simulink model "sound_effects"  (R2020b)
settings: Solver=FixedStepDiscrete  StartTime=0.0  StopTime=stopTime  RelTol=1e-3
PreLoadFcn:
  | addpath('../simple_gain_vector')
  | addpath('../flanger')
  | addpath('../bitcrusher')
  | addpath('../echo')
InitFcn:
  | initCallback
StopFcn:
  | stopCallback
undefined symbols (not defined in the file or in its folder): mp
settings Model: DataTypeOverride=Off  Creator=Ross  LastModifiedBy=wickh
settings SolverCC: AutoInsertRateTranBlk=on
settings DataIOCC: ReturnWorkspaceOutputs=off
settings OptimizationCC: BlockReduction=off  ConditionallyExecuteInputs=off  DefaultParameterBehavior=Inlined
settings DebuggingCC: SignalInfNanChecking=error  SignalRangeChecking=warning  ReadBeforeWriteMsg=DisableAll  WriteAfterWriteMsg=DisableAll  WriteAfterReadMsg=DisableAll  AlgebraicLoopMsg=error  MultiTaskDSMMsg=none  SingleTaskRateTransMsg=error  ParameterUnderflowMsg=warning  UnderSpecifiedDataTypeMsg=error  PregeneratedLibrarySubsystemCodeDiagnostic=none  ArithmeticOperatorsInVariantConditions=warning
settings HardwareCC: ProdBitPerPointer=32  ProdBitPerSizeT=32  ProdBitPerPtrDiffT=32  ProdLargestAtomicFloat=None  ProdIntDivRoundTo=Undefined  ProdEndianess=Unspecified  ProdWordSize=32  ProdHWDeviceType=ASIC/FPGA->ASIC/FPGA  TargetBitPerPointer=64  TargetBitPerSizeT=64  TargetBitPerPtrDiffT=64  TargetLongLongMode=on  TargetIntDivRoundTo=Zero  TargetEndianess=LittleEndian  TargetWordSize=64  TargetHWDeviceType=Custom Processor->MATLAB Host Computer  ProdEqTarget=off
settings ModelReferenceCC: UpdateModelReferenceTargets=IfOutOfDate
settings SFSimCC: SFSimEcho=off  SimUseLocalCustomCode=off  CustomCodeUndefinedFunction=UseInterfaceOnly
settings RTWCC: RTWUseLocalCustomCode=off

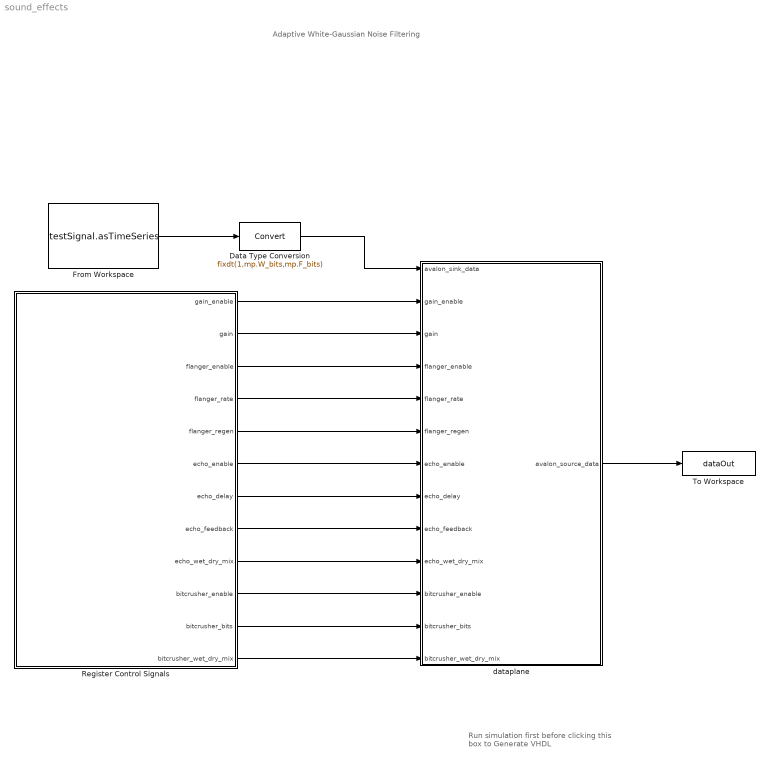
== system sound_effects ==
  note: Adaptive White-Gaussian Noise Filtering
  note: Run simulation first
      | before clicking this box to
      | Generate VHDL
  Data Type Conversion : DataTypeConversion  OutDataTypeStr=fixdt(1,mp.W_bits,mp.F_bits)
  From Workspace : FromWorkspace  VariableName=testSignal.asTimeSeries  OutDataTypeStr=double  SampleTime=mp.Ts_sim  Interpolate=off  OutputAfterFinalValue=Setting to zero
  Register Control Signals : Subsystem
  To Workspace : ToWorkspace  VariableName=dataOut  SaveFormat=Timeseries  SampleTime=-1
      settings: Save2DSignal=2-D array (concatenate along first dimension)
  dataplane : Subsystem  TreatAsAtomicUnit=on
  wires:
  dataplane/1(avalon_source_data) -> To Workspace/1
  From Workspace/1 -> Data Type Conversion/1
  Data Type Conversion/1 -> dataplane/1(avalon_sink_data)
  Register Control Signals/1(gain_enable) -> dataplane/2(gain_enable)
  Register Control Signals/2(gain) -> dataplane/3(gain)
  Register Control Signals/3(flanger_enable) -> dataplane/4(flanger_enable)
  Register Control Signals/4(flanger_rate) -> dataplane/5(flanger_rate)
  Register Control Signals/5(flanger_regen) -> dataplane/6(flanger_regen)
  Register Control Signals/6(echo_enable) -> dataplane/7(echo_enable)
  Register Control Signals/7(echo_delay) -> dataplane/8(echo_delay)
  Register Control Signals/8(echo_feedback) -> dataplane/9(echo_feedback)
  Register Control Signals/9(echo_wet_dry_mix) -> dataplane/10(echo_wet_dry_mix)
  Register Control Signals/10(bitcrusher_enable) -> dataplane/11(bitcrusher_enable)
  Register Control Signals/11(bitcrusher_bits) -> dataplane/12(bitcrusher_bits)
  Register Control Signals/12(bitcrusher_wet_dry_mix) -> dataplane/13(bitcrusher_wet_dry_mix)

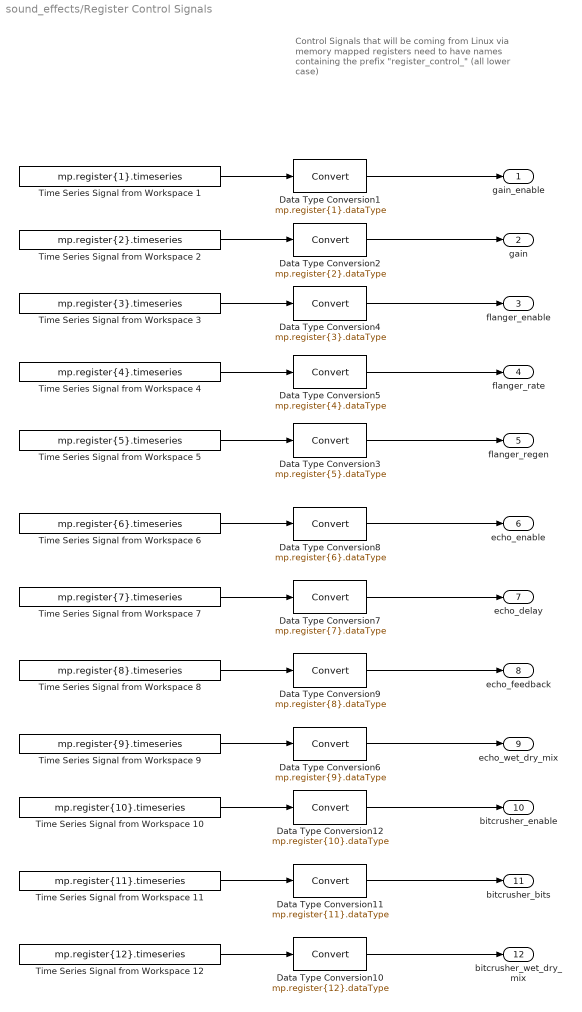
== system sound_effects/Register Control Signals ==
  note: Control Signals that will be coming from Linux via
      | memory mapped registers need to have names
      | containing the prefix "register_control_"
      | (all lower case)
  Data Type Conversion1 : DataTypeConversion  OutDataTypeStr=mp.register{1}.dataType
  Data Type Conversion10 : DataTypeConversion  OutDataTypeStr=mp.register{12}.dataType
  Data Type Conversion11 : DataTypeConversion  OutDataTypeStr=mp.register{11}.dataType
  Data Type Conversion12 : DataTypeConversion  OutDataTypeStr=mp.register{10}.dataType
  Data Type Conversion2 : DataTypeConversion  OutDataTypeStr=mp.register{2}.dataType
  Data Type Conversion3 : DataTypeConversion  OutDataTypeStr=mp.register{5}.dataType
  Data Type Conversion4 : DataTypeConversion  OutDataTypeStr=mp.register{3}.dataType
  Data Type Conversion5 : DataTypeConversion  OutDataTypeStr=mp.register{4}.dataType
  Data Type Conversion6 : DataTypeConversion  OutDataTypeStr=mp.register{9}.dataType
  Data Type Conversion7 : DataTypeConversion  OutDataTypeStr=mp.register{7}.dataType
  Data Type Conversion8 : DataTypeConversion  OutDataTypeStr=mp.register{6}.dataType
  Data Type Conversion9 : DataTypeConversion  OutDataTypeStr=mp.register{8}.dataType
  Time Series Signal from Workspace 1 : FromWorkspace  VariableName=mp.register{1}.timeseries  OutDataTypeStr=double  SampleTime=mp.Ts_sim
  Time Series Signal from Workspace 10 : FromWorkspace  VariableName=mp.register{10}.timeseries  OutDataTypeStr=double  SampleTime=mp.Ts_sim
  Time Series Signal from Workspace 11 : FromWorkspace  VariableName=mp.register{11}.timeseries  OutDataTypeStr=double  SampleTime=mp.Ts_sim
  Time Series Signal from Workspace 12 : FromWorkspace  VariableName=mp.register{12}.timeseries  OutDataTypeStr=double  SampleTime=mp.Ts_sim
  Time Series Signal from Workspace 2 : FromWorkspace  VariableName=mp.register{2}.timeseries  OutDataTypeStr=double  SampleTime=mp.Ts_sim
  Time Series Signal from Workspace 3 : FromWorkspace  VariableName=mp.register{3}.timeseries  OutDataTypeStr=double  SampleTime=mp.Ts_sim
  Time Series Signal from Workspace 4 : FromWorkspace  VariableName=mp.register{4}.timeseries  OutDataTypeStr=double  SampleTime=mp.Ts_sim
  Time Series Signal from Workspace 5 : FromWorkspace  VariableName=mp.register{5}.timeseries  OutDataTypeStr=double  SampleTime=mp.Ts_sim
  Time Series Signal from Workspace 6 : FromWorkspace  VariableName=mp.register{6}.timeseries  OutDataTypeStr=double  SampleTime=mp.Ts_sim
  Time Series Signal from Workspace 7 : FromWorkspace  VariableName=mp.register{7}.timeseries  OutDataTypeStr=double  SampleTime=mp.Ts_sim
  Time Series Signal from Workspace 8 : FromWorkspace  VariableName=mp.register{8}.timeseries  OutDataTypeStr=double  SampleTime=mp.Ts_sim
  Time Series Signal from Workspace 9 : FromWorkspace  VariableName=mp.register{9}.timeseries  OutDataTypeStr=double  SampleTime=mp.Ts_sim
  gain_enable : Outport  VectorParamsAs1DForOutWhenUnconnected=off
  gain : Outport  Port=2  VectorParamsAs1DForOutWhenUnconnected=off
  flanger_enable : Outport  Port=3  VectorParamsAs1DForOutWhenUnconnected=off
  flanger_rate : Outport  Port=4  VectorParamsAs1DForOutWhenUnconnected=off
  flanger_regen : Outport  Port=5  VectorParamsAs1DForOutWhenUnconnected=off
  echo_enable : Outport  Port=6  VectorParamsAs1DForOutWhenUnconnected=off
  echo_delay : Outport  Port=7  VectorParamsAs1DForOutWhenUnconnected=off
  echo_feedback : Outport  Port=8  VectorParamsAs1DForOutWhenUnconnected=off
  echo_wet_dry_mix : Outport  Port=9  VectorParamsAs1DForOutWhenUnconnected=off
  bitcrusher_enable : Outport  Port=10  VectorParamsAs1DForOutWhenUnconnected=off
  bitcrusher_bits : Outport  Port=11  VectorParamsAs1DForOutWhenUnconnected=off
  bitcrusher_wet_dry_mix : Outport  Port=12  VectorParamsAs1DForOutWhenUnconnected=off
  wires:
  Time Series Signal from Workspace 1/1 -> Data Type Conversion1/1
  Data Type Conversion1/1 -> gain_enable/1
  Time Series Signal from Workspace 2/1 -> Data Type Conversion2/1
  Data Type Conversion2/1 -> gain/1
  Data Type Conversion4/1 -> flanger_enable/1
  Data Type Conversion3/1 -> flanger_regen/1
  Data Type Conversion5/1 -> flanger_rate/1
  Time Series Signal from Workspace 5/1 -> Data Type Conversion3/1
  Time Series Signal from Workspace 3/1 -> Data Type Conversion4/1
  Time Series Signal from Workspace 4/1 -> Data Type Conversion5/1
  Data Type Conversion9/1 -> echo_feedback/1
  Data Type Conversion6/1 -> echo_wet_dry_mix/1
  Time Series Signal from Workspace 8/1 -> Data Type Conversion9/1
  Data Type Conversion8/1 -> echo_enable/1
  Time Series Signal from Workspace 9/1 -> Data Type Conversion6/1
  Data Type Conversion7/1 -> echo_delay/1
  Time Series Signal from Workspace 6/1 -> Data Type Conversion8/1
  Time Series Signal from Workspace 7/1 -> Data Type Conversion7/1
  Data Type Conversion12/1 -> bitcrusher_enable/1
  Time Series Signal from Workspace 10/1 -> Data Type Conversion12/1
  Time Series Signal from Workspace 12/1 -> Data Type Conversion10/1
  Data Type Conversion11/1 -> bitcrusher_bits/1
  Data Type Conversion10/1 -> bitcrusher_wet_dry_mix/1
  Time Series Signal from Workspace 11/1 -> Data Type Conversion11/1

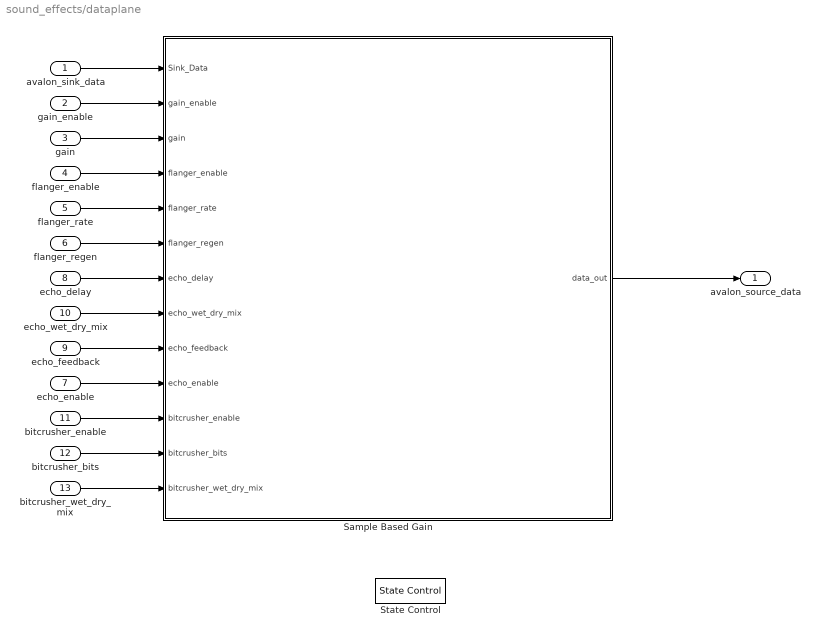
== system sound_effects/dataplane ==
  avalon_sink_data : Inport
  gain_enable : Inport  Port=2
  gain : Inport  Port=3
  flanger_enable : Inport  Port=4
  flanger_rate : Inport  Port=5
  flanger_regen : Inport  Port=6
  echo_enable : Inport  Port=7
  echo_delay : Inport  Port=8
  echo_feedback : Inport  Port=9
  echo_wet_dry_mix : Inport  Port=10
  bitcrusher_enable : Inport  Port=11
  bitcrusher_bits : Inport  Port=12
  bitcrusher_wet_dry_mix : Inport  Port=13
  Sample Based Gain : Subsystem
  State Control : StateControl  StateControl=Synchronous
  avalon_source_data : Outport  VectorParamsAs1DForOutWhenUnconnected=off
  wires:
  Sample Based Gain/1(data_out) -> avalon_source_data/1
  gain_enable/1 -> Sample Based Gain/2(gain_enable)
  avalon_sink_data/1 -> Sample Based Gain/1(Sink_Data)
  gain/1 -> Sample Based Gain/3(gain)
  flanger_enable/1 -> Sample Based Gain/4(flanger_enable)
  flanger_rate/1 -> Sample Based Gain/5(flanger_rate)
  flanger_regen/1 -> Sample Based Gain/6(flanger_regen)
  echo_feedback/1 -> Sample Based Gain/9(echo_feedback)
  echo_enable/1 -> Sample Based Gain/10(echo_enable)
  echo_wet_dry_mix/1 -> Sample Based Gain/8(echo_wet_dry_mix)
  echo_delay/1 -> Sample Based Gain/7(echo_delay)
  bitcrusher_enable/1 -> Sample Based Gain/11(bitcrusher_enable)
  bitcrusher_bits/1 -> Sample Based Gain/12(bitcrusher_bits)
  bitcrusher_wet_dry_mix/1 -> Sample Based Gain/13(bitcrusher_wet_dry_mix)

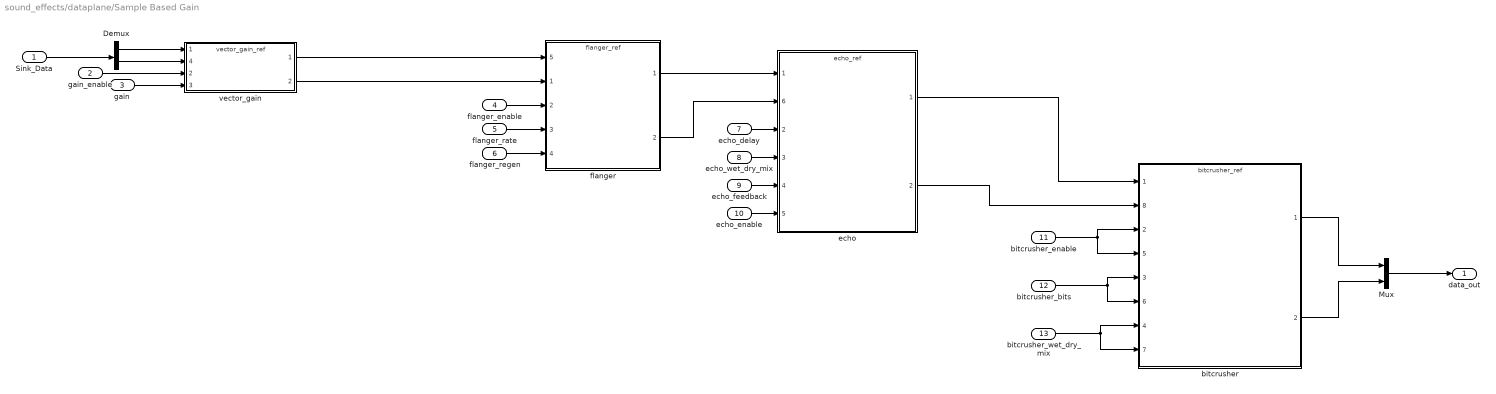
== system sound_effects/dataplane/Sample Based Gain ==
  Sink_Data : Inport
  gain_enable : Inport  Port=2
  gain : Inport  Port=3
  flanger_enable : Inport  Port=4
  flanger_rate : Inport  Port=5
  flanger_regen : Inport  Port=6
  echo_delay : Inport  Port=7
  echo_wet_dry_mix : Inport  Port=8
  echo_feedback : Inport  Port=9
  echo_enable : Inport  Port=10
  bitcrusher_enable : Inport  Port=11
  bitcrusher_bits : Inport  Port=12
  bitcrusher_wet_dry_mix : Inport  Port=13
  Demux : Demux  Outputs=2
  Mux : Mux  Inputs=2
  bitcrusher : ModelReference  ModelNameDialog=bitcrusher_ref  SimulationMode=Normal  ModelReferenceVersion=3.10
      settings: PortSchema="{\"entries\":[{\"content\":{\"sides\":[{\"content\":{\"connectorIds\":[\"In1\",\"In8\",\"In2\",\"In5\",\"In3\",\"In6\",\"In4\",\"In7\"]},\"type\":\"ConnectorPlacement.EquallySpacedRectSide\",\"uuid\":\"90c15296-b05c-4084-9131-8d1d83a85f81\"},{\"content\":{\"connectorIds\":[\"Out1\",\"Out2\"],\"side\":\"RIGHT\"},\"type\":\"ConnectorPlacement.EquallySpacedRectSide\",\"uuid\":\"9a8bffd3-a422-4815-8844-880c14b7d0b0\"},{\"content\":{\"connectorIds\":[],\"side\":\"TOP\"},\"type\":\"ConnectorPlacement.EquallySpacedRectSide\",\"uuid\":\"96339341-ea10-4881-8e29-794be7478c65\"},{\"content\":{\"connectorIds\":[],\"side\":\"HIDDEN\"},\"type\":\"ConnectorPlacement.EquallySpacedRectSide\",\"uuid\":\"4bb35bf2-de86-4de6-867a-84aa2bcf46f8\"}]},\"type\":\"ConnectorPlacement.EquallySpacedConnector\",\"uuid\":\"42256606-ddb3-4766-9977-bd7ae7f9f64f\"}],\"packageUris\":[\"http://schema.mathworks.com/mf0/Connector/R2020b\"],\"version\":\"1.0\"}"
  echo : ModelReference  ModelNameDialog=echo_ref  SimulationMode=Normal  ModelReferenceVersion=1.158
      settings: PortSchema="{\"entries\":[{\"content\":{\"sides\":[{\"content\":{\"connectorIds\":[\"In1\",\"In6\",\"In2\",\"In3\",\"In4\",\"In5\"]},\"type\":\"ConnectorPlacement.EquallySpacedRectSide\",\"uuid\":\"e306e1ad-d1b8-4582-952d-4c4191a99a81\"},{\"content\":{\"connectorIds\":[\"Out1\",\"Out2\"],\"side\":\"RIGHT\"},\"type\":\"ConnectorPlacement.EquallySpacedRectSide\",\"uuid\":\"8133f08a-39d0-44da-b52e-b96b1c72783c\"},{\"content\":{\"connectorIds\":[],\"side\":\"TOP\"},\"type\":\"ConnectorPlacement.EquallySpacedRectSide\",\"uuid\":\"327e31c7-8f91-4124-82a4-b2c62ce56765\"},{\"content\":{\"connectorIds\":[],\"side\":\"HIDDEN\"},\"type\":\"ConnectorPlacement.EquallySpacedRectSide\",\"uuid\":\"f85fe833-603d-4d04-9a61-60dde0930239\"}]},\"type\":\"ConnectorPlacement.EquallySpacedConnector\",\"uuid\":\"c6b2a458-4634-4ce8-98bc-50a2a0ff1bc4\"}],\"packageUris\":[\"http://schema.mathworks.com/mf0/Connector/R2020b\"],\"version\":\"1.0\"}"
  flanger : ModelReference  ModelNameDialog=flanger_ref  SimulationMode=Normal  ModelReferenceVersion=3.19
      settings: PortSchema="{\"entries\":[{\"content\":{\"sides\":[{\"content\":{\"connectorIds\":[\"In5\",\"In1\",\"In2\",\"In3\",\"In4\"]},\"type\":\"ConnectorPlacement.EquallySpacedRectSide\",\"uuid\":\"1d82ca4f-6eb6-4f28-946c-3ec85ec43cb1\"},{\"content\":{\"connectorIds\":[\"Out1\",\"Out2\"],\"side\":\"RIGHT\"},\"type\":\"ConnectorPlacement.EquallySpacedRectSide\",\"uuid\":\"239d2b31-0591-4f6b-b81b-3753802d9df9\"},{\"content\":{\"connectorIds\":[],\"side\":\"TOP\"},\"type\":\"ConnectorPlacement.EquallySpacedRectSide\",\"uuid\":\"6a0da88e-5604-41a7-848a-16d2caa5593e\"},{\"content\":{\"connectorIds\":[],\"side\":\"HIDDEN\"},\"type\":\"ConnectorPlacement.EquallySpacedRectSide\",\"uuid\":\"3b3b9426-683e-4311-a3c2-1e4479131ae9\"}]},\"type\":\"ConnectorPlacement.EquallySpacedConnector\",\"uuid\":\"3ff79b1b-4c7e-494f-b04d-fe3ab9f407cb\"}],\"packageUris\":[\"http://schema.mathworks.com/mf0/Connector/R2020b\"],\"version\":\"1.0\"}"
  vector_gain : ModelReference  ModelNameDialog=vector_gain_ref  SimulationMode=Normal  ModelReferenceVersion=1.247
      settings: PortSchema="{\"entries\":[{\"content\":{\"sides\":[{\"content\":{\"connectorIds\":[\"In1\",\"In4\",\"In2\",\"In3\"]},\"type\":\"ConnectorPlacement.EquallySpacedRectSide\",\"uuid\":\"8d28509a-bc74-4292-9a2c-b91be567764f\"},{\"content\":{\"connectorIds\":[\"Out1\",\"Out2\"],\"side\":\"RIGHT\"},\"type\":\"ConnectorPlacement.EquallySpacedRectSide\",\"uuid\":\"1dfc3807-3a0e-47fc-8f94-1ce52140c10f\"},{\"content\":{\"connectorIds\":[],\"side\":\"TOP\"},\"type\":\"ConnectorPlacement.EquallySpacedRectSide\",\"uuid\":\"39ce73be-d21d-426c-873d-5f452b093320\"},{\"content\":{\"connectorIds\":[],\"side\":\"HIDDEN\"},\"type\":\"ConnectorPlacement.EquallySpacedRectSide\",\"uuid\":\"45aa1cf0-577b-4409-a7ad-cf8e382955b5\"}]},\"type\":\"ConnectorPlacement.EquallySpacedConnector\",\"uuid\":\"e2f728cb-de10-4dce-913c-4d66a8425789\"}],\"packageUris\":[\"http://schema.mathworks.com/mf0/Connector/R2020b\"],\"version\":\"1.0\"}"
  data_out : Outport
  wires:
  gain_enable/1 -> vector_gain/2
  gain/1 -> vector_gain/3
  flanger/1 -> echo/1
  echo/1 -> bitcrusher/1
  flanger_enable/1 -> flanger/2
  flanger_rate/1 -> flanger/3
  flanger_regen/1 -> flanger/4
  echo_delay/1 -> echo/2
  echo_wet_dry_mix/1 -> echo/3
  echo_feedback/1 -> echo/4
  echo_enable/1 -> echo/5
  bitcrusher_enable/1 -> bitcrusher/2, bitcrusher/5
  bitcrusher_bits/1 -> bitcrusher/3, bitcrusher/6
  bitcrusher_wet_dry_mix/1 -> bitcrusher/4, bitcrusher/7
  Demux/2 -> vector_gain/4
  Sink_Data/1 -> Demux/1
  Demux/1 -> vector_gain/1
  vector_gain/1 -> flanger/5
  vector_gain/2 -> flanger/1
  echo/2 -> bitcrusher/8
  bitcrusher/1 -> Mux/1
  bitcrusher/2 -> Mux/2
  Mux/1 -> data_out/1
  flanger/2 -> echo/6
